simulink model "Contoller"  (R2020b)
settings: Solver=VariableStepAuto  StartTime=0.0  StopTime=10.0  RelTol=1e-3
settings Model: Creator=Xiao  LastModifiedBy=Xiao

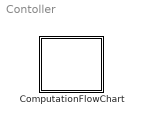
== system Contoller ==
  ComputationFlowChart : Stateflow chart  TreatAsAtomicUnit=on

== stateflow chart Contoller/ComputationFlowChart ==
  state Wait/
    % AXI4
    burst_start = 0;
    burst_length = 0;
    from_ddr_to_ram = 0;
    %PE
    PE_en = 0;
  state Idel/
  state Start/
    % AXI4
    burst_start = 0;
    burst_length = 0;
    from_ddr_to_ram = 0;
    %PE
    PE_en = 0;
  state Ex_Mem_RD/
    % AXI4
    burst_start = 1;
    burst_length = param_burst_length;
    from_ddr_to_ram = 1;
    %PE
    PE_en = 0;
  state Data_Convolution/
    %AXI4
    burst_start = 0;
    burst_length = param_burst_length;
    from_ddr_to_ram = 1;
    % PE
    PE_en = 1;
  state Ex_Men_WR/
    %AXI4
    burst_start = 1;
    burst_length = param_burst_length;
    from_ddr_to_ram = 0;
    %PE
    PE_en = 1;
  (default) -> Wait
  Wait -> Wait [order 2] : [ddr_init_done == 0]
  Wait -> Idel [order 1] : [ddr_init_done == 1]
  Idel -> Start
  Start -> Ex_Mem_RD
  Ex_Mem_RD -> Data_Convolution
  Data_Convolution -> Ex_Men_WR
